simulink model "dynamics_lab3"  (Simulink 8.0)
settings: Solver=ode1  StartTime=0.0  StopTime=1000  FixedStep=0.1  RelTol=1e-3
InitFcn:
  | clear all;close all;clc;warning off all;
settings Model: Creator=bleonard  LastModifiedBy=Grompone
settings DataIOCC: SignalLoggingSaveFormat=ModelDataLogs
settings OptimizationCC: InitFltsAndDblsToZero=on
settings DebuggingCC: SaveWithParameterizedLinksMsg=none  MultiTaskCondExecSysMsg=none  FcnCallInpInsideContextMsg=EnableAllAsWarning  StrictBusMsg=None
settings SFSimCC: SimParseCustomCode=off
settings RTWCC: IncludeERTFirstTime=on
settings GRTTargetCC: CombineOutputUpdateFcns=off  GRTInterface=on

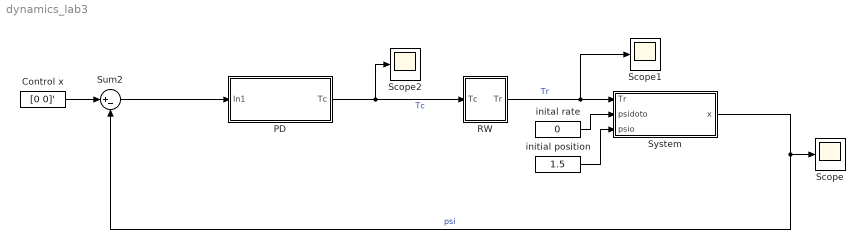
== system dynamics_lab3 ==
  Control x : Constant  Value=[0 0]'
  PD : Subsystem
  RW : Subsystem
  Scope : Scope
  Scope1 : Scope
  Scope2 : Scope
      settings: SaveName=ScopeData2
  Sum2 : Sum  Inputs=|+-  OutDataTypeStr=Inherit: Same as first input
  System : Subsystem
  inital rate : Constant  Value=0
  initial position : Constant  Value=1.5
  wires:
  PD/1(Tc) -> RW/1(Tc), Scope2/1  "Tc"
  RW/1(Tr) -> System/1(Tr), Scope1/1  "Tr"
  System/1(x) -> Scope/1, Sum2/2  "psi"
  Control x/1 -> Sum2/1
  inital rate/1 -> System/2(psidoto)
  initial position/1 -> System/3(psio)
  Sum2/1 -> PD/1(In1)

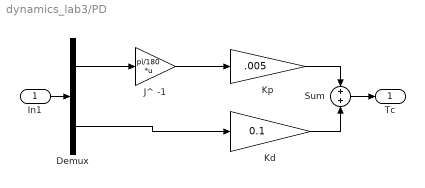
== system dynamics_lab3/PD ==
  In1 : Inport
  "   J^ -1" : Gain  Gain=pi/180  Multiplication=Matrix(K*u)  SaturateOnIntegerOverflow=on  OutDataTypeStr=Inherit: Same as input  ParamDataTypeStr=Inherit: Same as input
  Demux : Demux  Outputs=2
  Kd : Gain  Gain=0.1  OutDataTypeStr=Inherit: Same as input  ParamDataTypeStr=Inherit: Same as input
  Kp : Gain  Gain=.005  OutDataTypeStr=Inherit: Same as input  ParamDataTypeStr=Inherit: Same as input
  Sum : Sum  Inputs=+|+  OutDataTypeStr=Inherit: Same as first input
  Tc : Outport
  wires:
  In1/1 -> Demux/1
  Kp/1 -> Sum/1
  Kd/1 -> Sum/2
  Sum/1 -> Tc/1
  Demux/1 -> "   J^ -1"/1
  "   J^ -1"/1 -> Kp/1
  Demux/2 -> Kd/1

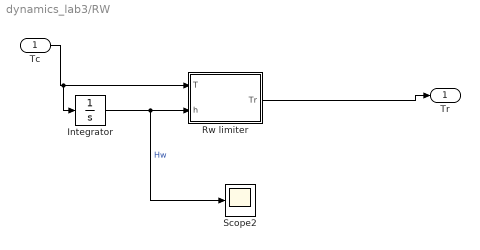
== system dynamics_lab3/RW ==
  Tc : Inport
  Integrator : Integrator
  Rw limiter : MATLAB Function  TreatAsAtomicUnit=on
  Scope2 : Scope
      settings: SaveName=ScopeData3
  Tr : Outport
  wires:
  Tc/1 -> Integrator/1, Rw limiter/1(T)
  Integrator/1 -> Rw limiter/2(h), Scope2/1  "Hw"
  Rw limiter/1(Tr) -> Tr/1

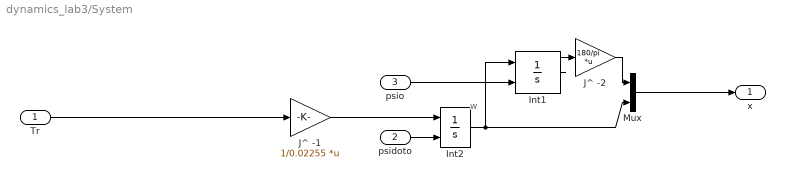
== system dynamics_lab3/System ==
  note: w
  Tr : Inport
  psidoto : Inport  Port=2
  psio : Inport  Port=3
  "   J^ -1" : Gain  Gain=1/0.02255  Multiplication=Matrix(K*u)  SaturateOnIntegerOverflow=on  OutDataTypeStr=Inherit: Same as input  ParamDataTypeStr=Inherit: Same as input
  "   J^ -2" : Gain  Gain=180/pi  Multiplication=Matrix(K*u)  SaturateOnIntegerOverflow=on  OutDataTypeStr=Inherit: Same as input  ParamDataTypeStr=Inherit: Same as input
  Int1 : Integrator  InitialConditionSource=external  InitialCondition=[0 0 -0.1]'
  Int2 : Integrator  InitialConditionSource=external  InitialCondition="[0  -0.001  0]'"
  Mux : Mux  Inputs=2
  x : Outport
  wires:
  Int2/1 -> Int1/1, Mux/2
  "   J^ -1"/1 -> Int2/1
  psidoto/1 -> Int2/2
  psio/1 -> Int1/2
  Mux/1 -> x/1
  Tr/1 -> "   J^ -1"/1
  Int1/1 -> "   J^ -2"/1
  "   J^ -2"/1 -> Mux/1

== matlab function RW/Rw limiter ==
  data: T input double; Tr output double; h input double
function Tr = fcn(T,h)
%#eml



hmax=.06; %absolute maximum momentum RW

Tmax=.005; %absolute maximum Torque RW



if abs(h)<hmax

if abs(T)>Tmax
    
    Trc=Tmax;
    
else
    
    Trc=abs(T);
    
end

else
    
  Trc=0;
  
end

Tr=sign(T)*Trc;
